simulink model "Transmitter"  (R2014a)
settings: Solver=ode45  StartTime=0.0  StopTime=0.5  RelTol=1e-3
values from neighbouring files (symbols this model uses):
  FrameTime = 3.2e-06    [Ofdm_Parameters.mat]
  qpsktxrxOFDM =     [Ofdm_Parameters.mat]
undefined symbols (not defined in the file or in its folder): Radix
libraries: dspsrcs4 x2, simulink x1, commcnvcod2 x1, commcrc2 x1, commblkintrlv2 x1, dspxfrm3 x1, commdigbbndam3 x1, commsdrhw_v2 x1
settings Model: Creator=root  LastModifiedBy=root

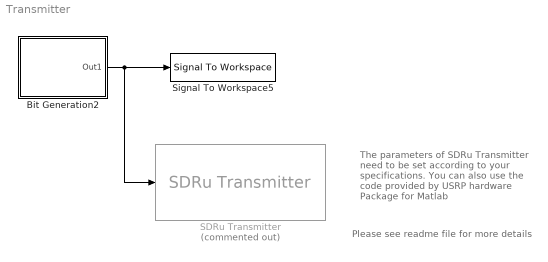
== system Transmitter ==
  note: Please see readme file for more details
  note: The parameters of SDRu Transmitter need to be set according to your specifications. You can also use the code provided by USRP hardware Package for Matlab
  Bit Generation2 : Subsystem
      mask Display: disp('TrAnSmItTeR')
  SDRu Transmitter : commsdrhw_v2/SDRu Transmitter  Commented=on  rxtx=tx  USRP2_IP='192.168.10.2'  centerFrequency=2.45e9  centerFrequencySrc=Dialog  loOffset=0  loOffsetSrc=Dialog  gain=8  gainSrc=Dialog  decimInterp=512  decimInterpSrc=Dialog  USRP2_IP_NUM=[49 57 50 46 49 54 56 46 49 48 46 50]  frameLength=362  outputDatatype=int16  overrunUnderrunPort=off  sampleTime=1  dboardInfo=|  HOST_DATA_PORT=30000  HOST_CONTROL_PORT=30001  USRP2_DATA_PORT=32769  USRP2_CONTROL_PORT=32768  bufferMode=Continuous streaming  EnableBurstMode=off  NumFramesInBurst=100
      | dbid: 0
      |           dbName: 'no db found'
      |          freqMin: 0
      |          freqMax: 0
      |          gainMin: 0
      |          gainMax: 0
      |     gainStepSize: 0
  Signal To Workspace5 : SignalToWorkspace  VariableName=final_TXData
      settings: CopyFcn=dspblkcopystw(gcbh);
  wires:
  Bit Generation2/1(Out1) -> SDRu Transmitter/1, Signal To Workspace5/1

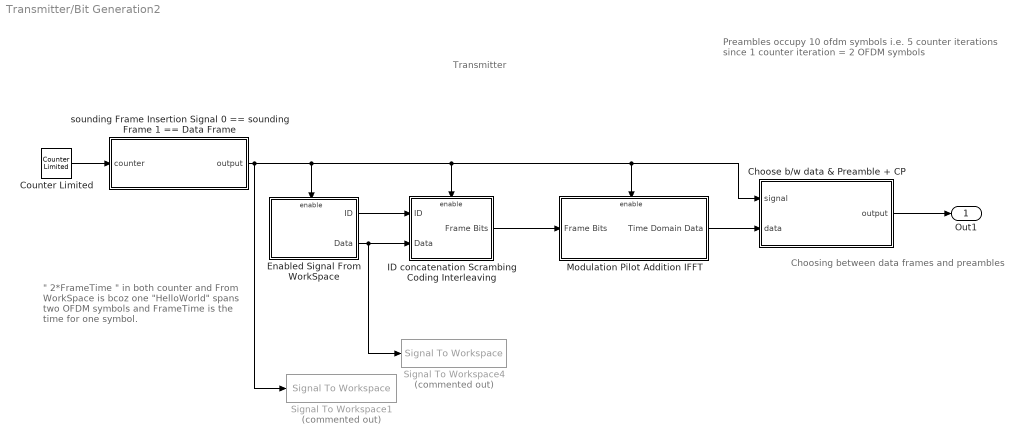
== system Transmitter/Bit Generation2 ==
  note: Choosing between data frames and preambles
  note: Preambles occupy 10 ofdm symbols i.e. 5 counter iterations
      | since 1 counter iteration = 2 OFDM symbols
  note: " 2*FrameTime " in  both counter and
      | From WorkSpace is bcoz one "HelloWorld"
      | spans two OFDM symbols and FrameTime
      | is the time for one symbol.
  note: Transmitter
  "Choose b/w data & Preamble + CP " : MATLAB Function
  Counter Limited : simulink/Sources/Counter Limited  uplimit=104  tsamp=2*FrameTime
  Enabled Signal From WorkSpace : Subsystem
  ID concatenation Scrambing Coding Interleaving : Subsystem
  Modulation Pilot Addition IFFT : Subsystem
  Signal To Workspace1 : SignalToWorkspace  Commented=on  VariableName=Signal_SoundingFrame
      settings: CopyFcn=dspblkcopystw(gcbh);
  Signal To Workspace4 : SignalToWorkspace  Commented=on  VariableName=triggeredData1
      settings: CopyFcn=dspblkcopystw(gcbh);  Save2DSignal=3-D array (concatenate along third dimension)
  sounding Frame Insertion Signal 0 == sounding Frame 1 == Data Frame : MATLAB Function  TreatAsAtomicUnit=on
  Out1 : Outport
  wires:
  Counter Limited/1 -> sounding Frame Insertion Signal 0 == sounding Frame 1 == Data Frame/1(counter)
  sounding Frame Insertion Signal 0 == sounding Frame 1 == Data Frame/1(output) -> ID concatenation Scrambing Coding Interleaving/Enable, Modulation Pilot Addition IFFT/Enable, "Choose b/w data & Preamble + CP "/1(signal), Enabled Signal From WorkSpace/Enable, Signal To Workspace1/1
  Enabled Signal From WorkSpace/2(Data) -> Signal To Workspace4/1, ID concatenation Scrambing Coding Interleaving/2(Data)
  Modulation Pilot Addition IFFT/1(Time Domain Data) -> "Choose b/w data & Preamble + CP "/2(data)
  "Choose b/w data & Preamble + CP "/1(output) -> Out1/1
  Enabled Signal From WorkSpace/1(ID) -> ID concatenation Scrambing Coding Interleaving/1(ID)
  ID concatenation Scrambing Coding Interleaving/1(Frame Bits) -> Modulation Pilot Addition IFFT/1(Frame Bits)

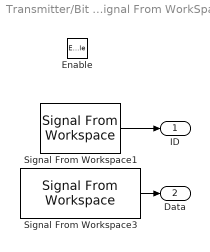
== system Transmitter/Bit Generation2/Enabled Signal From WorkSpace ==
  Enable : EnablePort
  Signal From Workspace1 : dspsrcs4/Signal From Workspace  X=ID  Ts=2*FrameTime/(qpsktxrxOFDM.IDLength)  nsamps=qpsktxrxOFDM.IDLength  OutputAfterFinalValue=Cyclic repetition  ignoreOrWarnInputAndFrameLengths=off
  Signal From Workspace3 : dspsrcs4/Signal From Workspace  X=qpsktxrxOFDM.sBit  Ts=2*FrameTime/(qpsktxrxOFDM.DataLength)  nsamps=qpsktxrxOFDM.DataLength  OutputAfterFinalValue=Cyclic repetition  ignoreOrWarnInputAndFrameLengths=off
  ID : Outport
  Data : Outport  Port=2
  wires:
  Signal From Workspace3/1 -> Data/1
  Signal From Workspace1/1 -> ID/1

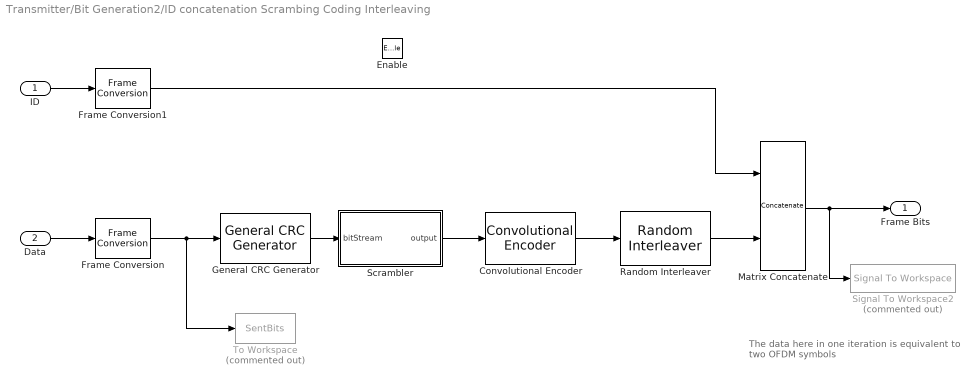
== system Transmitter/Bit Generation2/ID concatenation Scrambing Coding Interleaving ==
  note: The data here in one iteration is equivalent
      | to two OFDM symbols
  ID : Inport
  Data : Inport  Port=2
  Enable : EnablePort
  Convolutional Encoder : commcnvcod2/Convolutional Encoder  trellis=trellis  opMode=Truncated (reset every frame)  DelayedResetAction=off  hasIniStPort=off  hasFinStPort=off  usePuncVector=off  punctureVector=[1; 1; 0; 1; 0; 1]  reset=Unused parameter value
  Frame Conversion : FrameConversion  OutFrame=Sample-based
  Frame Conversion1 : FrameConversion  OutFrame=Sample-based
  General CRC Generator : commcrc2/General CRC Generator  genPoly=[1 0 0 0 0 0 0 0 1 1 1 1 1]  iniStates=0  directMethod=off  reflectInputBytes=off  reflectChecksums=off  finalXOR=0  numChecksums=1
  Matrix Concatenate : Concatenate  Mode=Multidimensional array
  Random Interleaver : commblkintrlv2/Random Interleaver  N=(qpsktxrxOFDM.DataLength + qpsktxrxOFDM.CRCLength ) * qpsktxrxOFDM.CodeRate  seed=12345
  Scrambler : MATLAB Function  TreatAsAtomicUnit=on
  Signal To Workspace2 : SignalToWorkspace  Commented=on  VariableName=SentLayeredBits
      settings: CopyFcn=dspblkcopystw(gcbh);  Save2DSignal=3-D array (concatenate along third dimension)
  To Workspace : ToWorkspace  Commented=on  VariableName=SentBits  SampleTime=-1
  Frame Bits : Outport
  wires:
  Frame Conversion/1 -> General CRC Generator/1, To Workspace/1
  Frame Conversion1/1 -> Matrix Concatenate/1
  Convolutional Encoder/1 -> Random Interleaver/1
  ID/1 -> Frame Conversion1/1
  Data/1 -> Frame Conversion/1
  Random Interleaver/1 -> Matrix Concatenate/2
  Matrix Concatenate/1 -> Frame Bits/1, Signal To Workspace2/1
  General CRC Generator/1 -> Scrambler/1(bitStream)
  Scrambler/1(output) -> Convolutional Encoder/1

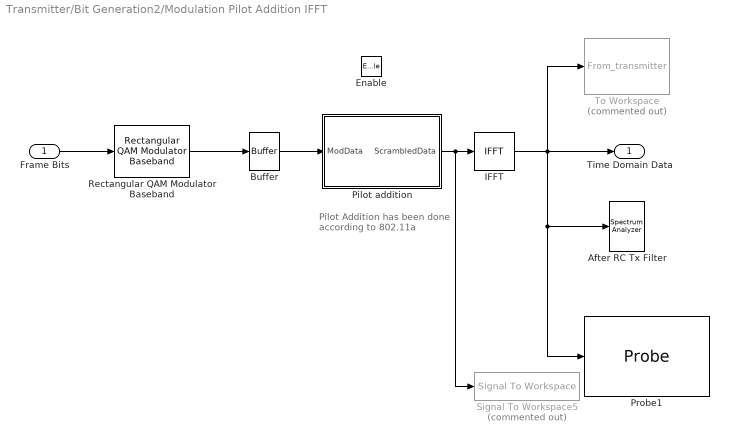
== system Transmitter/Bit Generation2/Modulation Pilot Addition IFFT ==
  note: Pilot Addition has been done
      | according to 802.11a
  Frame Bits : Inport
  Enable : EnablePort
  After RC Tx Filter : SpectrumAnalyzer
  Buffer : Buffer  N=qpsktxrxOFDM.NumDataSubCarriers  TreatMby1Signals=One channel
  IFFT : dspxfrm3/IFFT  CompMethod=Table lookup  TableOpt=NEW  TableOptActive=Speed  BitRevOrder=off  cs_in=off  SkipNorm=on  InheritFFTLength=on  FFTLength=64  WrapInput=on  mode=Complex  outSamplingMode=Sample based  RowConvenienceOn=on  FFTImplementation=Radix-2  firstCoeffDataTypeStr=Inherit: Same word length as input  firstCoeffLastDataTypeStr=Inherit: Same word length as input  outputMin=[]  outputMax=[]  roundingMode=Floor  overflowMode=off
  Pilot addition : MATLAB Function  TreatAsAtomicUnit=on
  Probe1 : Probe  ProbeComplexSignal=off
  Rectangular QAM Modulator Baseband : commdigbbndam3/Rectangular QAM Modulator Baseband  M=qpsktxrxOFDM.M  InType=Bit  Enc=Gray  Mapping=[0:15]  PowType=Average Power  MinDist=2  AvgPow=1  PeakPow=1  Ph=0  outDtype=double  outWordLen=16  outUDDataType=sfix(16)  outFracLenMode=Best precision  outFracLen=15
  Signal To Workspace5 : SignalToWorkspace  Commented=on  VariableName=TXData_freq
      settings: CopyFcn=dspblkcopystw(gcbh);
  To Workspace : ToWorkspace  Commented=on  VariableName=From_transmitter  SampleTime=-1
  Time Domain Data : Outport
  wires:
  IFFT/1 -> Time Domain Data/1, Probe1/1, After RC Tx Filter/1, To Workspace/1
  Frame Bits/1 -> Rectangular QAM Modulator Baseband/1
  Pilot addition/1(ScrambledData) -> Signal To Workspace5/1, IFFT/1
  Buffer/1 -> Pilot addition/1(ModData)
  Rectangular QAM Modulator Baseband/1 -> Buffer/1

== matlab function Transmitter/Bit Generation2/Choose b//w data & Preamble + CP  ==
  data: signal input; data input; output output; qpsktxrxOFDM parameter
function output = Choose_frame(signal , data , qpsktxrxOFDM)
% CHOOSING DATA FRAMES AND SOUNDING FRAMES. THE NUMBER OF DATA FRAMES
% BETWEEN TWO SOUNDING FRAMES ARE SELECTED FROM "COUNTER LIMITED" BLOCK IN
% SIMULINK
persistent i ;

if isempty(i)
   i = 1;
end


output = complex(zeros(80,1));

if signal == 1          % DATA %

    output = [data(49:64); data];
    i = 1;
    
elseif signal == 0                    % Preambles %
   
    output = qpsktxrxOFDM.Preamble(i : i + 79);
    i = i + 80;
    
end


end

== matlab function Transmitter/Bit Generation2/ID concatenation Scrambing Coding Interleaving/Scrambler ==
  data: bitStream input; output output
function output = scrambler(bitStream)
% performs scrambing according to wifi 802.11
persistent state;

if isempty(state)
   state = [1 0 1 1 1 0 1];
end

bitLength = 174 + 12;   %length + CRC

output = zeros(bitLength,1);
poly = state;

for i = 1:bitLength
    output(i) = mod(poly(1) + poly(4) , 2);
    poly = [poly(2:end) output(i)];
end

output = mod(output + bitStream , 2 );

state = poly;


end

== matlab function Transmitter/Bit Generation2/Modulation Pilot Addition IFFT/Pilot addition ==
  data: ModData input; ScrambledData output
function ScrambledData   = pilotAddition( ModData)

persistent state;

if isempty(state)
   state = [1 1 1 1 1 1 0];     % actual initial =  [1 1 1 1 1 1 1] but for skipping signal packet i evaluate first iteration by hand
end

bitLength = 1;

pilot = zeros(bitLength,1);
poly = state;

for i = 1:bitLength
    pilot(i) = mod(poly(1) + poly(4) , 2);
    poly = [poly(2:end) pilot(i)];
end

if pilot == 0
    pilot = 1;
elseif pilot == 1
    pilot = -1;
end    
    
state = poly;

completeDatatemp = complex(zeros(1,53));
completeDatatemp(1:5) = ModData(1:5);
completeDatatemp(6) = 1*pilot;                  %pilot                    
completeDatatemp(7:19) = ModData(6:18);
completeDatatemp(20) = 1*pilot;
completeDatatemp(21:26) = ModData(19:24);
completeDatatemp(27) = 0;
completeDatatemp(28:33) = ModData(25:30);
completeDatatemp(34) = 1*pilot;
completeDatatemp(35:47) = ModData(31:43);
completeDatatemp(48) = -1*pilot;
completeDatatemp(49:53) = ModData(44:48);

% persistent p;
% if isempty(p)
%     p = 0;
% end
%     p = p+1;
% 
% completeDatatemp = complex(zeros(1,53));
% completeDatatemp(1:5) = ModData(1:5);
% completeDatatemp(6) = 1*p;                  %pilot                    
% completeDatatemp(7:19) = ModData(6:18);
% completeDatatemp(20) = 1*p;
% completeDatatemp(21:26) = ModData(19:24);
% completeDatatemp(27) = 0;
% completeDatatemp(28:33) = ModData(25:30);
% completeDatatemp(34) = 1*p;
% completeDatatemp(35:47) = ModData(31:43);
% completeDatatemp(48) = -1*p;
% completeDatatemp(49:53) = ModData(44:48);

completeData = complex(zeros(1,64));
completeData(7:59) = completeDatatemp;
completeData = fftshift(completeData);          % subcarrier arrangement : 0 , 1 , 2 .......63

ScrambledData = complex(zeros(64,1));
ScrambledData = completeData.';

return;

end

== matlab function Transmitter/Bit Generation2/sounding Frame Insertion Signal 0 == sounding Frame 1 == Data Frame ==
  data: counter input; output output
function output   = soundingFrameInsertion( counter )

output = 1;
 
if (counter < 5)
    output = 0;
end

% if mod(counter , 2) == 0
%     output = 1;
% end
% 
% if counter < 2 
%     output = 0;
% end

end
